simulink model "HIL"  (R2023a)
settings: Solver=FixedStepAuto  StartTime=0.0  StopTime=inf  RelTol=1e-3  EnableMultiTasking=on
values from neighbouring files (symbols this model uses):
  k = temp    [Calculations.m]
libraries: simulink_extras x4, arduinolib x3, simulink x1
settings Model: ExtModeTrigDuration=2  Creator=youss  LastModifiedBy=youss
settings OptimizationCC: EnhancedBackFolding=on  PassReuseOutputArgsAs=Individual arguments  ZeroExternalMemoryAtStartup=off  ZeroInternalMemoryAtStartup=off  MaxStackSize=64  OptimizeBlockOrder=speed  DifferentSizesBufferReuse=on  OptimizationCustomize=off  EfficientTunableParamExpr=on
settings DebuggingCC: ParameterTunabilityLossMsg=error
settings HardwareCC: ProdBitPerInt=16  ProdBitPerPointer=16  ProdBitPerSizeT=16  ProdBitPerPtrDiffT=16  ProdLargestAtomicFloat=None  ProdWordSize=8  ProdHWDeviceType=Atmel->AVR
settings SFSimCC: MATLABDynamicMemAlloc=off
settings RTWCC: Description=Embedded Coder  SystemTargetFile=ert.tlc  HardwareBoard=Arduino Uno  TemplateMakefile=ert_default_tmf  Toolchain=Arduino AVR  BuildConfiguration=Faster Runs
settings CodeAppCC: ForceParamTrailComments=on  IgnoreCustomStorageClasses=off  OperatorAnnotations=on  SimulinkDataObjDesc=on  SFDataObjDesc=on  InsertBlockDesc=on
settings ERTTargetCC: SupportContinuousTime=on  SupportVariableSizeSignals=on  ExtModeTransport=3  ExtModeStaticAlloc=on  ExtModeAutomaticAllocSize=off  ExtModeStaticAllocSize=250  ExtModeMexFile=ext_xcp  ExtModeIntrfLevel=Level2 - Open

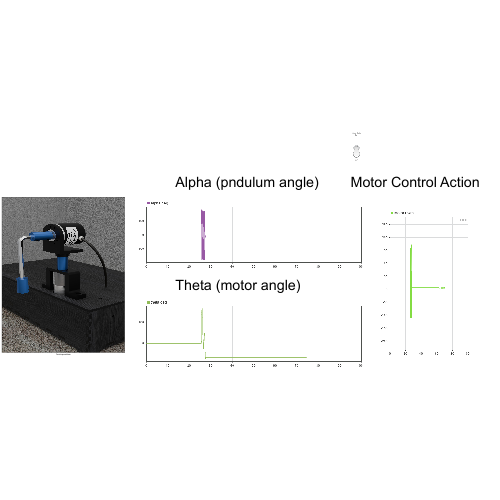
[thumbnail: Simulink's stored preview of the top-level diagram]
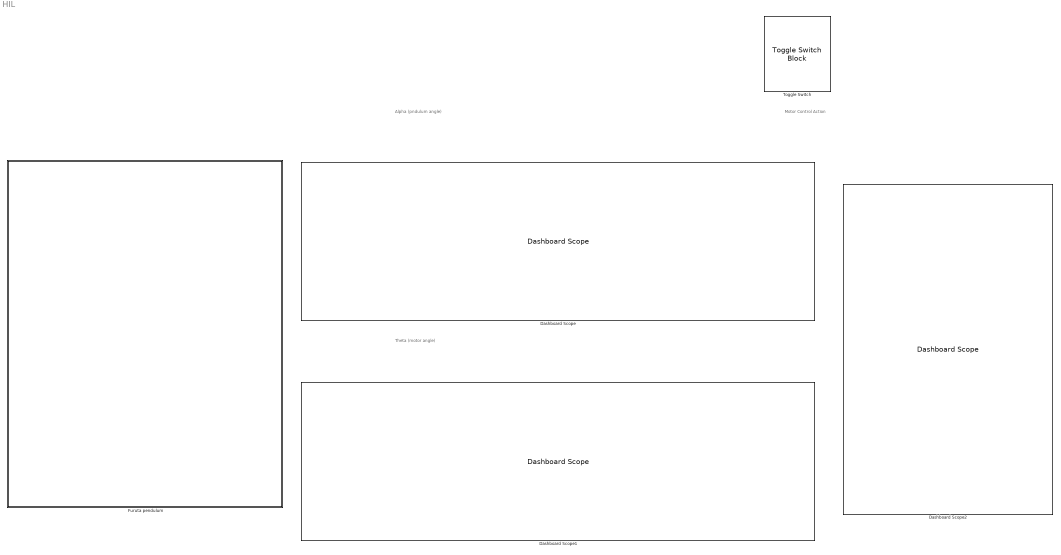
== system HIL ==
  note: Alpha (pndulum angle)
  note: Theta (motor angle)
  note: Motor Control Action
  Dashboard Scope : DashboardScope  Ymin=-185  Ymax=185
  Dashboard Scope1 : DashboardScope  Ymin=-185  Ymax=185
  Dashboard Scope2 : DashboardScope  Ymin=-13  Ymax=13
  Furuta pendulum : Subsystem
      mask Display: image('5.jpg'); % Use "Edit Image" on toolstrip to change.
  Toggle Switch : ToggleSwitchBlock
      settings: Values={{'Off', 'On'}, [0 1]}

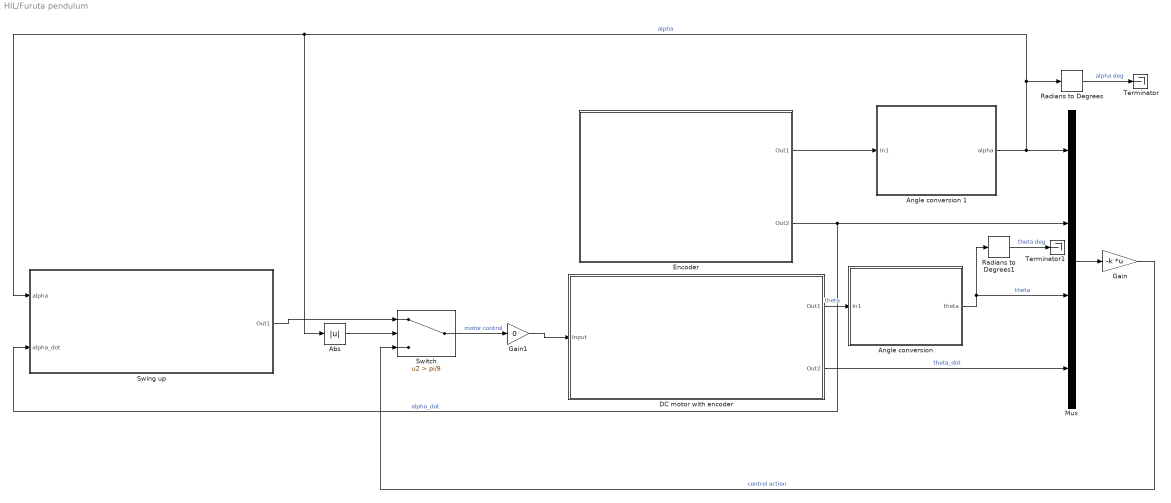
== system HIL/Furuta pendulum ==
  Abs : Abs  SaturateOnIntegerOverflow=off
  Angle conversion : Subsystem
  Angle conversion 1 : Subsystem
  DC motor with encoder : Subsystem
      mask Display: image('NFP-JGA25-370-EN-small-dc-gear-motors-with-encoder.png'); % Use "Edit Image" on toolstrip to change.
  Encoder : Subsystem
      mask Display: image('Encoder.png'); % Use "Edit Image" on toolstrip to change.
  Gain : Gain  Gain=-k  Multiplication=Matrix(K*u)
  Gain1 : Gain  Gain=0
  Mux : Mux
  Radians to Degrees : simulink_extras/Transformations/Radians to Degrees
  Radians to Degrees1 : simulink_extras/Transformations/Radians to Degrees
  Swing up : Subsystem
  Switch : Switch  Criteria=u2 > Threshold  Threshold=pi/9  SaturateOnIntegerOverflow=off  InputSameDT=off
  Terminator : Terminator
  Terminator1 : Terminator
  wires:
  Encoder/1(Out1) -> Angle conversion 1/1(In1)
  Gain/1 -> Switch/3  "control action"
  Encoder/2(Out2) -> Swing up/2(alpha_dot), Mux/2  "alpha_dot"
  Angle conversion 1/1(alpha) -> Swing up/1(alpha), Abs/1, Radians to Degrees/1, Mux/1  "alpha"
  Switch/1 -> Gain1/1  "motor control"
  Mux/1 -> Gain/1
  Angle conversion/1(theta) -> Mux/3, Radians to Degrees1/1  "theta"
  DC motor with encoder/2(Out2) -> Mux/4  "theta_dot"
  Radians to Degrees1/1 -> Terminator1/1  "theta deg"
  Abs/1 -> Switch/2
  DC motor with encoder/1(Out1) -> Angle conversion/1(In1)  "theta"
  Radians to Degrees/1 -> Terminator/1  "alpha deg"
  Swing up/1(Out1) -> Switch/1
  Gain1/1 -> DC motor with encoder/1(Input)

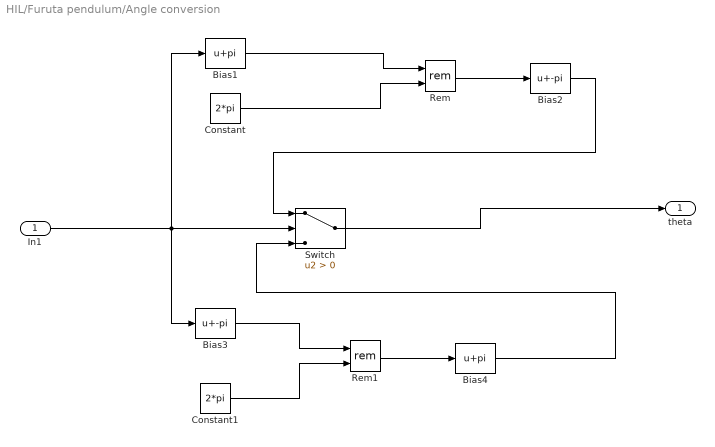
== system HIL/Furuta pendulum/Angle conversion ==
  In1 : Inport
  Bias1 : Bias  Bias=pi  SaturateOnIntegerOverflow=off
  Bias2 : Bias  Bias=-pi  SaturateOnIntegerOverflow=off
  Bias3 : Bias  Bias=-pi  SaturateOnIntegerOverflow=off
  Bias4 : Bias  Bias=pi  SaturateOnIntegerOverflow=off
  Constant : Constant  Value=2*pi
  Constant1 : Constant  Value=2*pi
  Rem : Math  Operator=rem
  Rem1 : Math  Operator=rem
  Switch : Switch  Criteria=u2 > Threshold  SaturateOnIntegerOverflow=off  InputSameDT=off
  theta : Outport
  wires:
  Bias4/1 -> Switch/3
  Bias3/1 -> Rem1/1
  Rem1/1 -> Bias4/1
  Switch/1 -> theta/1
  Bias1/1 -> Rem/1
  Constant/1 -> Rem/2
  In1/1 -> Switch/2, Bias1/1, Bias3/1
  Rem/1 -> Bias2/1
  Bias2/1 -> Switch/1
  Constant1/1 -> Rem1/2

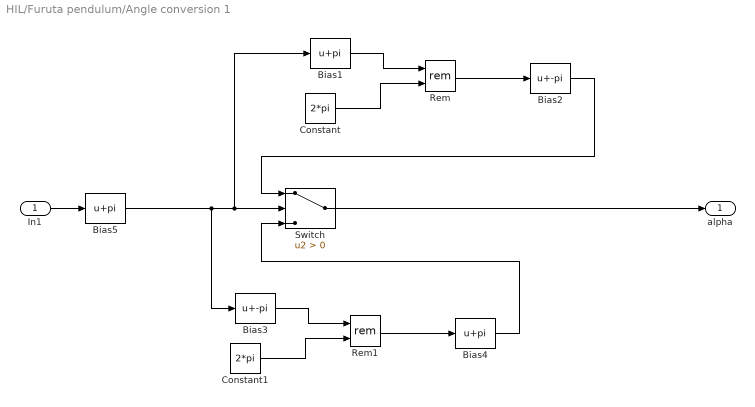
== system HIL/Furuta pendulum/Angle conversion 1 ==
  In1 : Inport
  Bias1 : Bias  Bias=pi  SaturateOnIntegerOverflow=off
  Bias2 : Bias  Bias=-pi  SaturateOnIntegerOverflow=off
  Bias3 : Bias  Bias=-pi  SaturateOnIntegerOverflow=off
  Bias4 : Bias  Bias=pi  SaturateOnIntegerOverflow=off
  Bias5 : Bias  Bias=pi  SaturateOnIntegerOverflow=off
  Constant : Constant  Value=2*pi
  Constant1 : Constant  Value=2*pi
  Rem : Math  Operator=rem
  Rem1 : Math  Operator=rem
  Switch : Switch  Criteria=u2 > Threshold  SaturateOnIntegerOverflow=off  InputSameDT=off
  alpha : Outport
  wires:
  Bias5/1 -> Switch/2, Bias1/1, Bias3/1
  Bias1/1 -> Rem/1
  Constant/1 -> Rem/2
  In1/1 -> Bias5/1
  Rem/1 -> Bias2/1
  Rem1/1 -> Bias4/1
  Constant1/1 -> Rem1/2
  Bias3/1 -> Rem1/1
  Switch/1 -> alpha/1
  Bias2/1 -> Switch/1
  Bias4/1 -> Switch/3

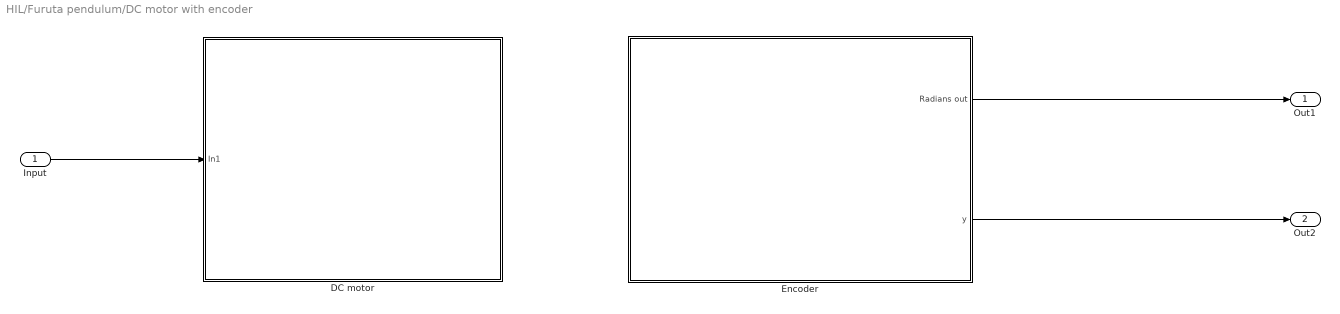
== system HIL/Furuta pendulum/DC motor with encoder ==
  Input : Inport
  DC motor : Subsystem
      mask Display: image('41gfmLvsoqL._AC_UF894,1000_QL80_.jpg'); % Use "Edit Image" on toolstrip to change.
  Encoder : Subsystem
      mask Display: image('m encoder.jpg'); % Use "Edit Image" on toolstrip to change.
  Out1 : Outport
  Out2 : Outport  Port=2
  wires:
  Input/1 -> DC motor/1(In1)
  Encoder/1(Radians out) -> Out1/1
  Encoder/2(y) -> Out2/1

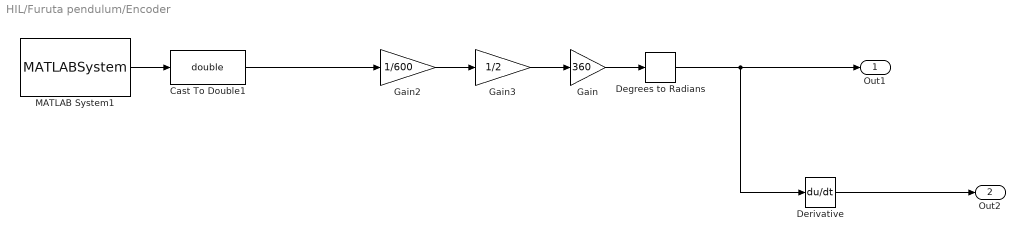
== system HIL/Furuta pendulum/Encoder ==
  Cast To Double1 : DataTypeConversion  OutDataTypeStr=double  SaturateOnIntegerOverflow=off  RndMeth=Floor
  Degrees to Radians : simulink_extras/Transformations/Degrees to Radians
  Derivative : Derivative
  Gain : Gain  Gain=360
  Gain2 : Gain  Gain=1/600
  Gain3 : Gain  Gain=1/2
  MATLAB System1 : MATLABSystem  System=Encoder_arduino  Encoder=0  PinA=2  PinB=4  SampleTime=0.01
      mask Type: Encoder_arduino
      mask Display:
      | disp('Encoder');
      | port_label('output',1,'y');
  Out1 : Outport
  Out2 : Outport  Port=2
  wires:
  Gain2/1 -> Gain3/1
  Gain3/1 -> Gain/1
  Cast To Double1/1 -> Gain2/1
  MATLAB System1/1 -> Cast To Double1/1
  Derivative/1 -> Out2/1
  Gain/1 -> Degrees to Radians/1
  Degrees to Radians/1 -> Derivative/1, Out1/1

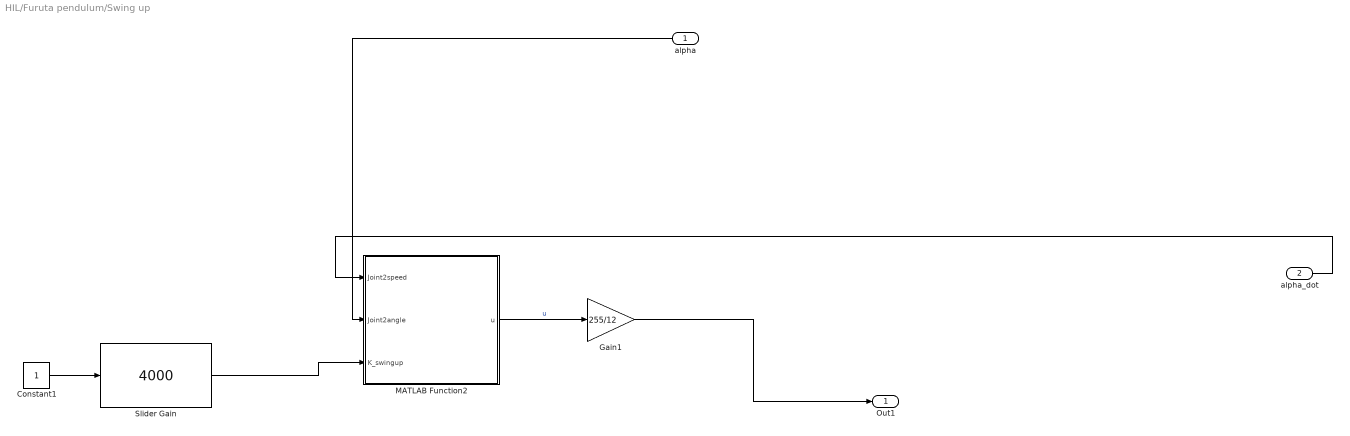
== system HIL/Furuta pendulum/Swing up ==
  alpha : Inport
  alpha_dot : Inport  Port=2
  Constant1 : Constant
  Gain1 : Gain  Gain=255/12
  MATLAB Function2 : MATLAB Function  TreatAsAtomicUnit=on
  Slider Gain : simulink/Math Operations/Slider Gain  gain=4000  low=0  high=10000
  Out1 : Outport
  wires:
  MATLAB Function2/1(u) -> Gain1/1  "u"
  alpha/1 -> MATLAB Function2/2(Joint2angle)
  Gain1/1 -> Out1/1
  Slider Gain/1 -> MATLAB Function2/3(K_swingup)
  Constant1/1 -> Slider Gain/1
  alpha_dot/1 -> MATLAB Function2/1(Joint2speed)

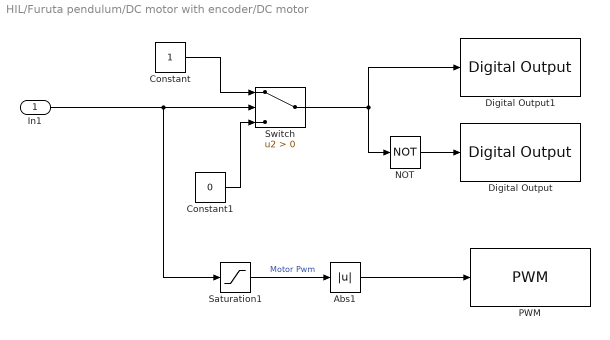
== system HIL/Furuta pendulum/DC motor with encoder/DC motor ==
  In1 : Inport
  Abs1 : Abs  SaturateOnIntegerOverflow=off
  Constant : Constant
  Constant1 : Constant  Value=0
  Digital Output : arduinolib/Digital Output  pinNumber=7  Direction=output  blockPlatform=arduino
  Digital Output1 : arduinolib/Digital Output  pinNumber=8  Direction=output  blockPlatform=arduino
  NOT : Logic  Operator=NOT  IconShape=distinctive  AllPortsSameDT=off  OutDataTypeStr=boolean
  PWM : arduinolib/PWM  pinNumber=11  frequencyType=Default  desiredFrequency=490.2  achievableFrequency=490.2
  Saturation1 : Saturate  UpperLimit=255  LowerLimit=-255
  Switch : Switch  Criteria=u2 > Threshold  SaturateOnIntegerOverflow=off  InputSameDT=off
  wires:
  Switch/1 -> NOT/1, Digital Output1/1
  In1/1 -> Saturation1/1, Switch/2
  Constant/1 -> Switch/1
  Constant1/1 -> Switch/3
  Abs1/1 -> PWM/1
  NOT/1 -> Digital Output/1
  Saturation1/1 -> Abs1/1  "Motor Pwm"

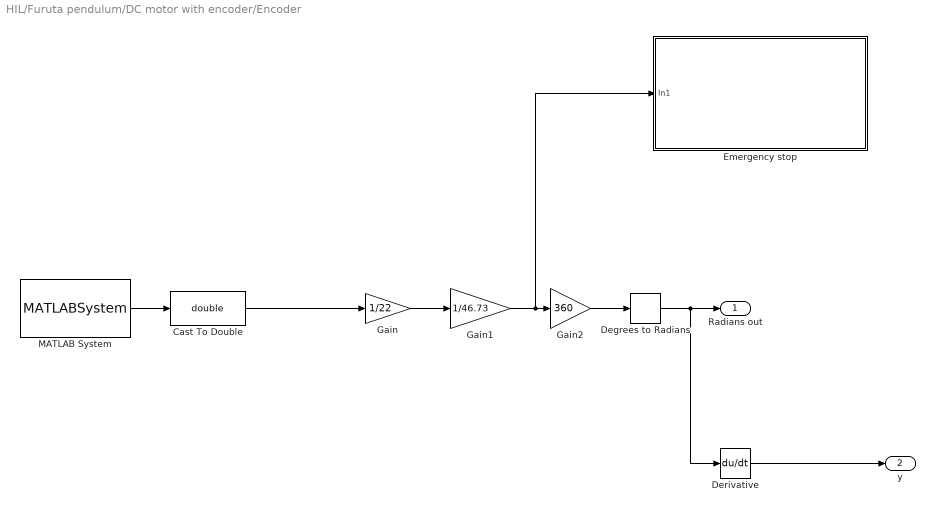
== system HIL/Furuta pendulum/DC motor with encoder/Encoder ==
  Cast To Double : DataTypeConversion  OutDataTypeStr=double  SaturateOnIntegerOverflow=off  RndMeth=Floor
  Degrees to Radians : simulink_extras/Transformations/Degrees to Radians
  Derivative : Derivative
  Emergency stop : Subsystem
      mask Display: image('Emergency stop.jpg'); % Use "Edit Image" on toolstrip to change.
  Gain : Gain  Gain=1/22
  Gain1 : Gain  Gain=1/46.73
  Gain2 : Gain  Gain=360
  MATLAB System : MATLABSystem  System=Encoder_arduino  Encoder=1  PinA=3  PinB=5  SampleTime=0.01
      mask Type: Encoder_arduino
      mask Display:
      | disp('Encoder');
      | port_label('output',1,'y');
  Radians out : Outport
  y : Outport  Port=2
  wires:
  Degrees to Radians/1 -> Derivative/1, Radians out/1
  Cast To Double/1 -> Gain/1
  MATLAB System/1 -> Cast To Double/1
  Gain/1 -> Gain1/1
  Gain2/1 -> Degrees to Radians/1
  Derivative/1 -> y/1
  Gain1/1 -> Emergency stop/1(In1), Gain2/1

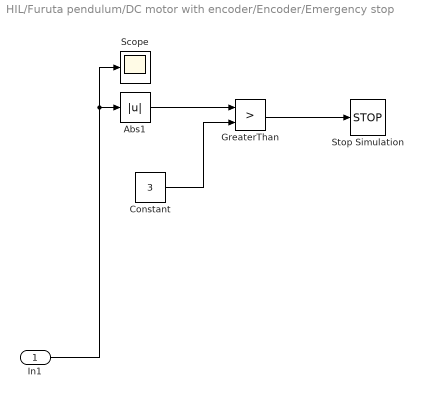
== system HIL/Furuta pendulum/DC motor with encoder/Encoder/Emergency stop ==
  In1 : Inport
  Abs1 : Abs  SaturateOnIntegerOverflow=off
  Constant : Constant  Value=3
  GreaterThan : RelationalOperator  Operator=>  OutDataTypeStr=boolean  RndMeth=Simplest  InputSameDT=off
  Scope : Scope
  Stop Simulation : Stop
  wires:
  GreaterThan/1 -> Stop Simulation/1
  Abs1/1 -> GreaterThan/1
  In1/1 -> Scope/1, Abs1/1
  Constant/1 -> GreaterThan/2

== matlab function HIL/Furuta pendulum/Swing up/MATLAB Function2 ==
  data: Joint2speed input; u output; Joint2angle input; K_swingup input
function u = fcn(Joint2speed,Joint2angle,K_swingup)

i=1;
g = 9.81;
m=0.010143116119298235; %Kg
I=5.7375077224929614*1e-6; %Kg.m^2
l=27.156641173388582*1e-3; %[m]

if Joint2angle>2*pi
    Joint2angle = Joint2angle-(2*pi);
elseif Joint2angle < 0
    Joint2angle = Joint2angle +2*pi;
end

S=sign(Joint2speed*cos(Joint2angle));

if Joint2speed * cos(Joint2angle) >=0
    delta=1;
else
    delta=-1;
end


E = 0.5*(I+m*l^2)*Joint2speed^2 + m*g*l*(cos(Joint2angle)-1);
E_norm =E/(m*g*l);
E_ref = 0;
E_err = E_ref-E;

u = K_swingup*(E_err)*delta;

% if Joint2speed ==0
%     i=i+1;
% end
% if mod(i,2)
%     u = K_swingup*E_err*delta;
% else
%     u = -K_swingup*E_err*delta;
% end
if Joint2angle <=(pi/11) && Joint2angle >=-(pi/11)
    u =0;
end
end
